simulink model "Ultrasonic"  (R2022b)
settings: Solver=ode4  StartTime=0.0  StopTime=inf  FixedStep=0.01  RelTol=1e-3  EnableMultiTasking=on
libraries: arduinolib x4, simulink x2, arduinosensorlib x1
settings Model: ExtModeTrigDuration=2  Creator=user  LastModifiedBy=user
settings DataIOCC: ReturnWorkspaceOutputs=off
settings OptimizationCC: EnhancedBackFolding=on  PassReuseOutputArgsAs=Individual arguments  ZeroExternalMemoryAtStartup=off  ZeroInternalMemoryAtStartup=off  MaxStackSize=64  OptimizeBlockOrder=speed  DifferentSizesBufferReuse=on  OptimizationCustomize=off  EfficientTunableParamExpr=on
settings DebuggingCC: ParameterTunabilityLossMsg=error
settings HardwareCC: ProdBitPerInt=16  ProdBitPerPointer=16  ProdBitPerSizeT=16  ProdBitPerPtrDiffT=16  ProdLargestAtomicFloat=None  ProdWordSize=8  ProdHWDeviceType=Atmel->AVR
settings SFSimCC: MATLABDynamicMemAlloc=off
settings RTWCC: Description=Embedded Coder  SystemTargetFile=ert.tlc  HardwareBoard=Arduino Mega 2560  TLCOptions=-aInlineSetEventsForThisBaseRateFcn=TLC_FALSE -aSuppressMultiTaskScheduler=TLC_FALSE -aRateBasedStepFcn=1  TemplateMakefile=ert_default_tmf  Toolchain=Arduino AVR  BuildConfiguration=Faster Runs
settings CodeAppCC: ForceParamTrailComments=on  IgnoreCustomStorageClasses=off  OperatorAnnotations=on  SimulinkDataObjDesc=on  SFDataObjDesc=on  InsertBlockDesc=on
settings ERTTargetCC: SupportContinuousTime=on  SupportVariableSizeSignals=on  ExtModeTransport=3  ExtModeStaticAlloc=on  ExtModeAutomaticAllocSize=off  ExtModeStaticAllocSize=2048  ExtModeMexFile=ext_xcp  ExtModeIntrfLevel=Level2 - Open

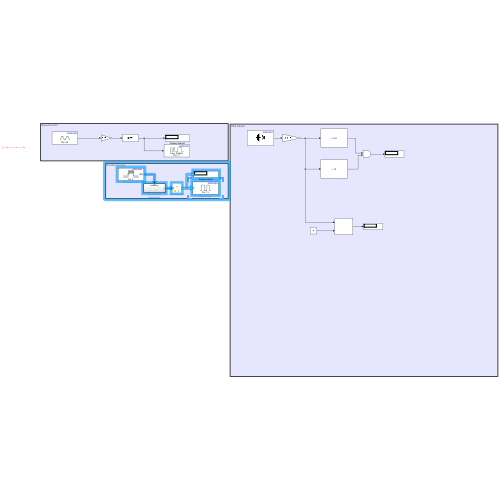
[thumbnail: Simulink's stored preview of the top-level diagram]
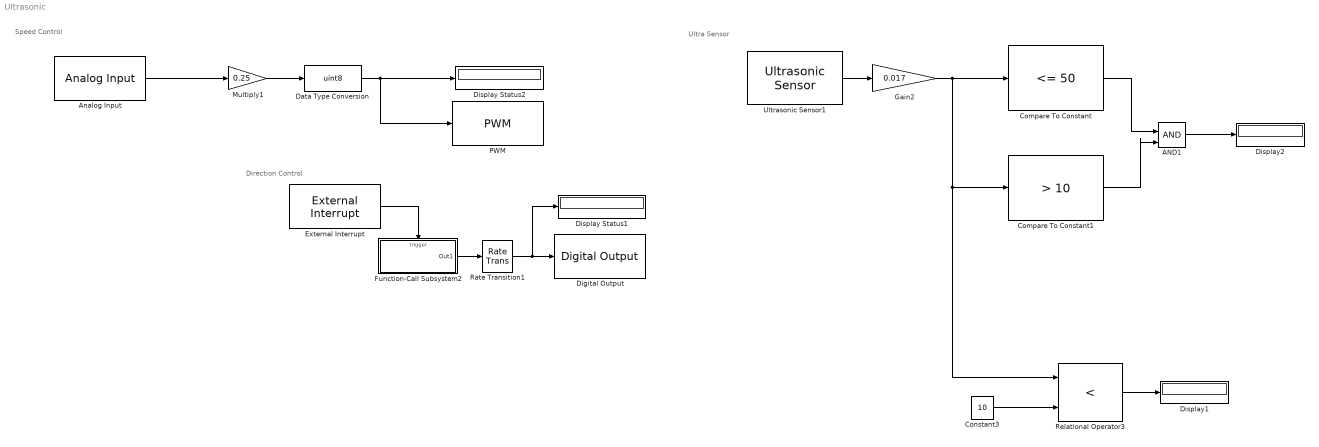
== system Ultrasonic ==
  note: Ultra Sensor
  note: Direction Control
  note: Speed Control
  AND1 : Logic  IconShape=distinctive  AllPortsSameDT=off  OutDataTypeStr=boolean
  Analog Input : arduinolib/Analog Input  pinNumber=0  ReadResultsOnly=off  ConversionTriggerSource=Software  ExternalTriggerType=uint32( 0 )  OutputDataType=uint16  EnableConversionCompleteNotify=off  EnableOuputStatus=off  SampleTime=-1  blockPlatform=arduino
  Compare To Constant : simulink/Logic and Bit Operations/Compare To Constant  relop=<=  const=50  OutDataTypeStr=boolean
  Compare To Constant1 : simulink/Logic and Bit Operations/Compare To Constant  relop=>  const=10  OutDataTypeStr=boolean
  Constant3 : Constant  Value=10
  Data Type Conversion : DataTypeConversion  OutDataTypeStr=uint8  SaturateOnIntegerOverflow=off  RndMeth=Floor
  Digital Output : arduinolib/Digital Output  pinNumber=13  Direction=output  blockPlatform=arduino
  Display Status1 : Display
  Display Status2 : Display
  Display1 : Display
  Display2 : Display
  External Interrupt : arduinolib/External Interrupt  Pin=2  PullUp=off  Mode=FALLING  InterruptSimulationInput=off
  Function-Call Subsystem2 : Subsystem  TreatAsAtomicUnit=on
  Gain2 : Gain  Gain=0.017
  Multiply1 : Gain  Gain=0.25
  PWM : arduinolib/PWM  pinNumber=11  frequencyType=Default  desiredFrequency=490.2  achievableFrequency=490.2
  Rate Transition1 : RateTransition  Deterministic=off
  Relational Operator3 : RelationalOperator  Operator=<  OutDataTypeStr=boolean  RndMeth=Simplest  InputSameDT=off
  Ultrasonic Sensor1 : arduinosensorlib/Ultrasonic Sensor  NumSignalPins=2  TrigPin=50  EchoPin=51  SignalPin=3  SampleTime_=0.1  blockPlatform=ARDUINO
  wires:
  ? -> ?
  Analog Input/1 -> Multiply1/1
  Compare To Constant/1 -> AND1/1
  Multiply1/1 -> Data Type Conversion/1
  Gain2/1 -> Compare To Constant/1, Compare To Constant1/1, Relational Operator3/1
  Compare To Constant1/1 -> AND1/2
  Ultrasonic Sensor1/1 -> Gain2/1
  Constant3/1 -> Relational Operator3/2
  Rate Transition1/1 -> Display Status1/1, Digital Output/1
  AND1/1 -> Display2/1
  External Interrupt/1 -> Function-Call Subsystem2/Trigger
  Relational Operator3/1 -> Display1/1
  Function-Call Subsystem2/1(Out1) -> Rate Transition1/1
  Data Type Conversion/1 -> PWM/1, Display Status2/1

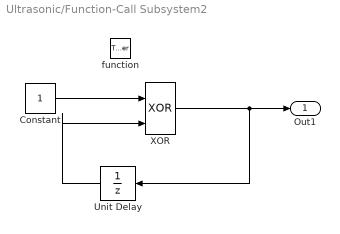
== system Ultrasonic/Function-Call Subsystem2 ==
  function : TriggerPort  TriggerType=function-call  VariantControl=(inherit)
  Constant : Constant
  Unit Delay : UnitDelay  SampleTime=-1  HasFrameUpgradeWarning=on
  XOR : Logic  Operator=XOR  IconShape=distinctive  AllPortsSameDT=off  OutDataTypeStr=boolean
  Out1 : Outport
  wires:
  Constant/1 -> XOR/1
  Unit Delay/1 -> XOR/2
  XOR/1 -> Unit Delay/1, Out1/1
